simulink model "closedloopwithvariableinput"  (R2016a)
settings: Solver=VariableStepAuto  StartTime=0.0  StopTime=10.0  RelTol=1e-3
libraries: arduinolib x4, dspadpt3 x1
settings Model: Creator=dell  LastModifiedBy=dell

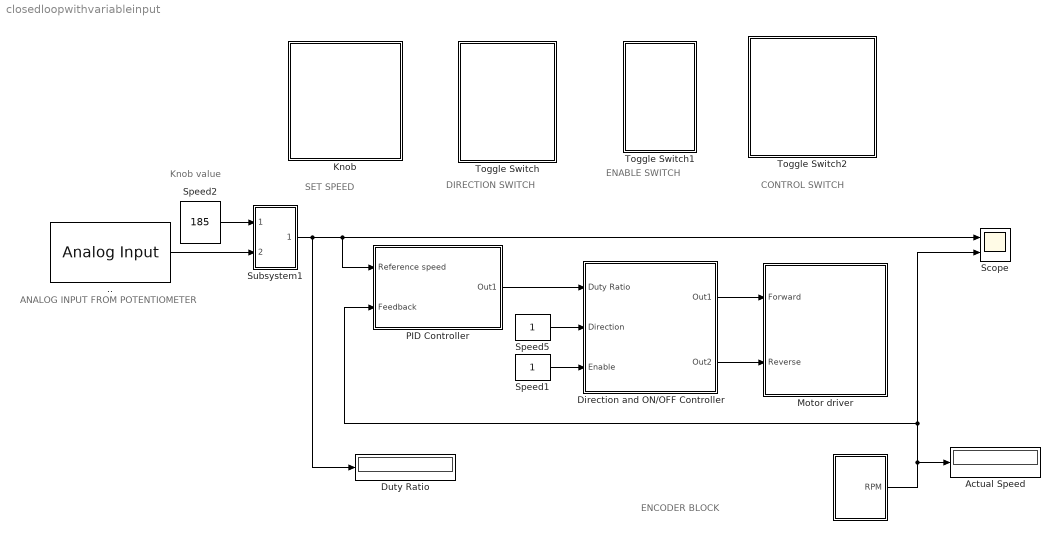
== system closedloopwithvariableinput ==
  note: DIRECTION SWITCH
  note: ANALOG INPUT
      | FROM POTENTIOMETER
  note: SET SPEED
  note: Knob value
  note: ENABLE SWITCH
  note: CONTROL SWITCH
  note: ENCODER BLOCK
  " " : Subsystem
  .. : arduinolib/Analog Input  pinNumber=0  sampleTime=0.001  blockPlatform=arduino
  Actual Speed : Display
  Direction and ON/OFF Controller : Subsystem
  Duty Ratio : Display
  Knob : Subsystem  DialogController=hmiCreateDDGDialog  IsWebBlock=on  mask(MWDashboardBlock){webBlockId=bad20c72-3a81-465b-aca1-27ab5a06c83c, webBlockType=continuousknob, ShowInLibBrowser=on, ShowInitialText=on, HMISrcModelName=untitled}
      mask prompts: webBlockId "WebBlock Id"; webBlockType "WebBlock Type"; HMISrcModelName "Source Model"
      mask Help: helpview([docroot '/mapfiles/simulink.map'], 'hmi_knob')
      mask Display:
      | if strcmp(get_param(bdroot(gcb),'BlockDiagramType'), 'library')
      |     image([(matlabroot) '/toolbox/simulink/hmi/icons/ContinuousKnob.png']);
      | end
  Motor driver : Subsystem
  PID Controller : Subsystem
  Scope : Scope  NumInputPorts=2
  Speed1 : Constant  OutMin=0  OutMax=100  OutDataTypeStr=single  SampleTime=0.001
  Speed2 : Constant  Value=185  OutMin=0  OutMax=250  OutDataTypeStr=single  SampleTime=0.001
  Speed5 : Constant  OutMin=0  OutMax=100  OutDataTypeStr=single  SampleTime=0.001
  Subsystem1 : Subsystem
  Toggle Switch : Subsystem  DialogController=hmiCreateDDGDialog  IsWebBlock=on  mask(MWDashboardBlock){webBlockId=f6c8166b-2cab-402f-842a-ce216d7d2c82, webBlockType=toggleswitch, ShowInLibBrowser=on, ShowInitialText=on, HMISrcModelName=untitled}
      mask prompts: webBlockId "WebBlock Id"; webBlockType "WebBlock Type"; HMISrcModelName "Source Model"
      mask Help: helpview([docroot '/mapfiles/simulink.map'], 'hmi_toggle_switch')
      mask Display:
      | if strcmp(get_param(bdroot(gcb),'BlockDiagramType'), 'library')
      |     image([(matlabroot) '/toolbox/simulink/hmi/icons/ToggleSwitch.png']);
      | end
  Toggle Switch1 : Subsystem  DialogController=hmiCreateDDGDialog  IsWebBlock=on  mask(MWDashboardBlock){webBlockId=53eccea4-bc18-4898-a6d0-165afc14bbde, webBlockType=toggleswitch, ShowInLibBrowser=on, ShowInitialText=on, HMISrcModelName=untitled}
      mask prompts: webBlockId "WebBlock Id"; webBlockType "WebBlock Type"; HMISrcModelName "Source Model"
      mask Help: helpview([docroot '/mapfiles/simulink.map'], 'hmi_toggle_switch')
      mask Display:
      | if strcmp(get_param(bdroot(gcb),'BlockDiagramType'), 'library')
      |     image([(matlabroot) '/toolbox/simulink/hmi/icons/ToggleSwitch.png']);
      | end
  Toggle Switch2 : Subsystem  DialogController=hmiCreateDDGDialog  IsWebBlock=on  mask(MWDashboardBlock){webBlockId=440d2440-ac7f-4a66-99f1-7b530808b111, webBlockType=toggleswitch, ShowInLibBrowser=on, ShowInitialText=on, HMISrcModelName=untitled}
      mask prompts: webBlockId "WebBlock Id"; webBlockType "WebBlock Type"; HMISrcModelName "Source Model"
      mask Help: helpview([docroot '/mapfiles/simulink.map'], 'hmi_toggle_switch')
      mask Display:
      | if strcmp(get_param(bdroot(gcb),'BlockDiagramType'), 'library')
      |     image([(matlabroot) '/toolbox/simulink/hmi/icons/ToggleSwitch.png']);
      | end
  wires:
  Speed5/1 -> Direction and ON/OFF Controller/2(Direction)
  Direction and ON/OFF Controller/1(Out1) -> Motor driver/1(Forward)
  Direction and ON/OFF Controller/2(Out2) -> Motor driver/2(Reverse)
  Speed1/1 -> Direction and ON/OFF Controller/3(Enable)
  " "/1(RPM) -> PID Controller/2(Feedback), Scope/2, Actual Speed/1
  Subsystem1/1(Out1) -> PID Controller/1(Reference speed), Scope/1, Duty Ratio/1
  Speed2/1 -> Subsystem1/1(In1)
  ../1 -> Subsystem1/2(In2)
  PID Controller/1(Out1) -> Direction and ON/OFF Controller/1(Duty Ratio)

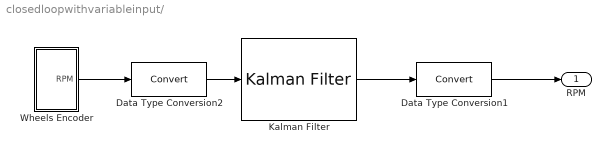
== system closedloopwithvariableinput/  ==
  " Wheels Encoder" : Subsystem  AncestorBlock=closedloop/Right Wheels Encoder
  Data Type Conversion1 : DataTypeConversion
  Data Type Conversion2 : DataTypeConversion
  Kalman Filter : dspadpt3/Kalman Filter  num_targets=1  sourceEnable=Always  isReset=on  X=zeros([1])  P=10*eye(1)  A=[1]  sourceMeasure=Specify via Dialog  H=[1]  Q=0.0005*eye(1)  R=eye(1)  isOutputEstMeasure=on  isOutputEstState=off  isOutputEstError=off  isOutputPrdMeasure=off  isOutputPrdState=off  isOutputPrdError=off
  RPM : Outport
  wires:
  " Wheels Encoder"/1(RPM) -> Data Type Conversion2/1
  Data Type Conversion2/1 -> Kalman Filter/1
  Kalman Filter/1 -> Data Type Conversion1/1
  Data Type Conversion1/1 -> RPM/1

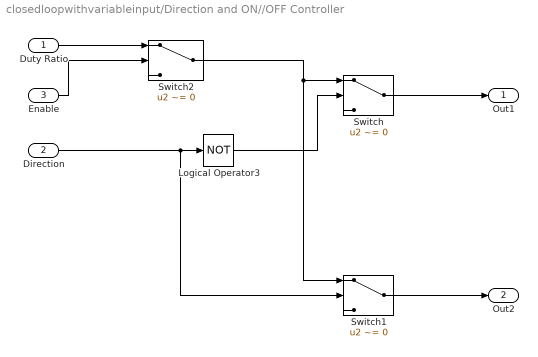
== system closedloopwithvariableinput/Direction and ON//OFF Controller ==
  Duty Ratio : Inport
  Direction : Inport  Port=2
  Enable : Inport  Port=3
  Logical Operator3 : Logic  Operator=NOT  AllPortsSameDT=off  OutDataTypeStr=boolean
  Switch : Switch  Criteria=u2 ~= 0
  Switch1 : Switch  Criteria=u2 ~= 0
  Switch2 : Switch  Criteria=u2 ~= 0
  Out1 : Outport
  Out2 : Outport  Port=2
  wires:
  Direction/1 -> Switch1/2, Logical Operator3/1
  Switch/1 -> Out1/1
  Switch1/1 -> Out2/1
  Duty Ratio/1 -> Switch2/1
  Enable/1 -> Switch2/2
  Switch2/1 -> Switch1/1, Switch/1
  Logical Operator3/1 -> Switch/2

== system closedloopwithvariableinput/Knob ==

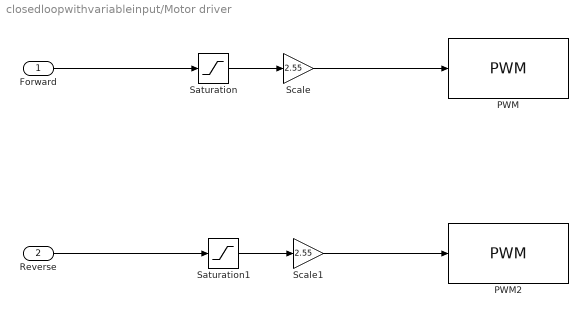
== system closedloopwithvariableinput/Motor driver ==
  Forward : Inport
  Reverse : Inport  Port=2
  PWM : arduinolib/PWM  pinNumber=5  blockPlatform=arduino
  PWM2 : arduinolib/PWM  pinNumber=4  blockPlatform=arduino
  Saturation : Saturate  UpperLimit=100  LowerLimit=0
      settings: AttributesFormatString=max = %<UpperLimit>\nmin = %<LowerLimit>
  Saturation1 : Saturate  UpperLimit=100  LowerLimit=0
      settings: AttributesFormatString=max = %<UpperLimit>\nmin = %<LowerLimit>
  Scale : Gain  Gain=2.55
  Scale1 : Gain  Gain=2.55
  wires:
  Saturation1/1 -> Scale1/1
  Scale1/1 -> PWM2/1
  Forward/1 -> Saturation/1
  Reverse/1 -> Saturation1/1
  Scale/1 -> PWM/1
  Saturation/1 -> Scale/1

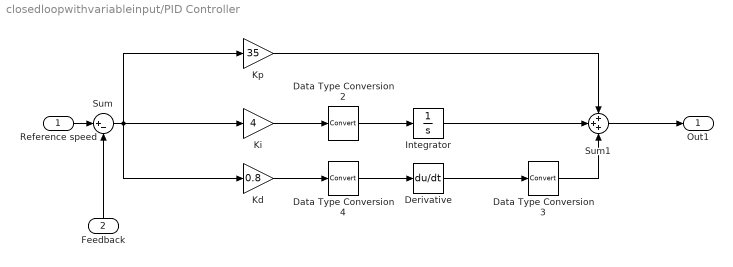
== system closedloopwithvariableinput/PID Controller ==
  Reference speed : Inport
  Feedback : Inport  Port=2
  Data Type Conversion2 : DataTypeConversion
  Data Type Conversion3 : DataTypeConversion
  Data Type Conversion4 : DataTypeConversion
  Derivative : Derivative
  Integrator : Integrator
  Kd : Gain  Gain=0.8
  Ki : Gain  Gain=4
  Kp : Gain  Gain=35
  Sum : Sum  Inputs=|+-
  Sum1 : Sum  Inputs=+++
  Out1 : Outport
  wires:
  Reference speed/1 -> Sum/1
  Feedback/1 -> Sum/2
  Kp/1 -> Sum1/1
  Ki/1 -> Data Type Conversion2/1
  Integrator/1 -> Sum1/2
  Kd/1 -> Data Type Conversion4/1
  Sum/1 -> Ki/1, Kp/1, Kd/1
  Data Type Conversion2/1 -> Integrator/1
  Data Type Conversion4/1 -> Derivative/1
  Derivative/1 -> Data Type Conversion3/1
  Sum1/1 -> Out1/1
  Data Type Conversion3/1 -> Sum1/3

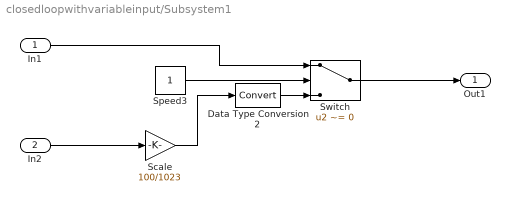
== system closedloopwithvariableinput/Subsystem1 ==
  In1 : Inport
  In2 : Inport  Port=2
  Data Type Conversion2 : DataTypeConversion
  Scale : Gain  Gain=100/1023
  Speed3 : Constant  OutMin=0  OutMax=100  OutDataTypeStr=single  SampleTime=0.001
  Switch : Switch  Criteria=u2 ~= 0
  Out1 : Outport
  wires:
  Speed3/1 -> Switch/2
  Scale/1 -> Data Type Conversion2/1
  Switch/1 -> Out1/1
  Data Type Conversion2/1 -> Switch/3
  In2/1 -> Scale/1
  In1/1 -> Switch/1

== system closedloopwithvariableinput/Toggle Switch ==

== system closedloopwithvariableinput/Toggle Switch1 ==

== system closedloopwithvariableinput/Toggle Switch2 ==

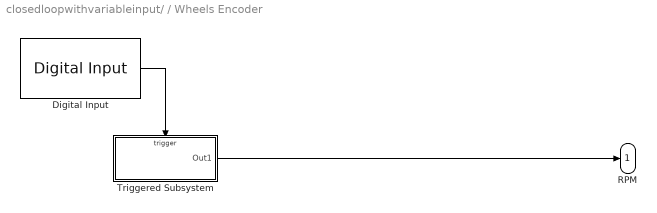
== system closedloopwithvariableinput/ / Wheels Encoder ==
  Digital Input : arduinolib/Digital Input  pinNumber=2  sampleTime=0.001  blockPlatform=arduino
  Triggered Subsystem : Subsystem  TreatAsAtomicUnit=on
  RPM : Outport
  wires:
  Digital Input/1 -> Triggered Subsystem/Trigger
  Triggered Subsystem/1(Out1) -> RPM/1

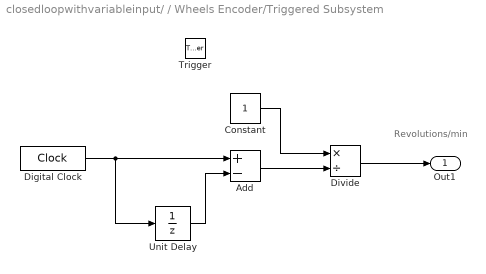
== system closedloopwithvariableinput/ / Wheels Encoder/Triggered Subsystem ==
  note: Revolutions/min
  Trigger : TriggerPort  VariantControl=Variant
  Add : Sum  Inputs=+-
  Constant : Constant
  Digital Clock : DigitalClock  SampleTime=-1
  Divide : Product  Inputs=*/  OutDataTypeStr=int32
  Unit Delay : UnitDelay  SampleTime=-1
  Out1 : Outport
  wires:
  Constant/1 -> Divide/1
  Divide/1 -> Out1/1
  Add/1 -> Divide/2
  Unit Delay/1 -> Add/2
  Digital Clock/1 -> Unit Delay/1, Add/1
